simulink model "Model_10_1"  (R2021a)
settings: Solver=VariableStepAuto  StartTime=0.0  StopTime=10  RelTol=1e-3
InitFcn:
  | bx=25; %25
  | bl=50; %50
  | bc=0.1; %0.08
  | 
  | ml=2; %2
  | 
  | mc=0.5;
  | M2=0.5;
  | 
  | mt=5;
  | g=9.81;
  | l_ref=0.3; %0.3
  | l_ini=1;   %1
  | l=l_ini;
  | x_ref=1; %3
  | n1=1; %5
  | n2=1;
  | 
  | L_2=0;  %chieu dai day nang ha
  | 
  | theta1_ini=0*pi/180;
  | theta2_ini=0*pi/180;  %2*pi/180
  | 
  | L_tai=0.1;
  | %ADRC' s parameter caculation
  | %b0 = (1)/(mc+mt+ml);
  | b0=(ml+mc)/(mt*mc+2*ml*mc+mt*ml+ml^2+mc^2); %Enhanced-coupling
  | %k_ESO = 100;
  | k_ESO = 100;
  | T_set  = 3; %5;
  | 
  | s_cl = -5.85/T_set;
  | Kp   = s_cl^2;
  | Kd   = -2*s_cl;
  | 
  | s_ESO = k_ESO*s_cl;
  | l1        = -3*s_ESO;
  | l2        = 3*( s_ESO)^2;
  | l3        = -(s_ESO)^3;
  | 
  | %b1 = (mt+mc)/(mc*ml +mc*mt+ml*mt);
  | b1=1/(ml+mc);
  | k_ESO1 =100; %100
  | T_set1  = 3;   %3
  | s_cl1 = -5.85/T_set1;
  | Kp1   = s_cl1^2;
  | Kd1   = -2*s_cl1;
  | 
  | s_ESO1 = k_ESO1*s_cl1;
  | l11        = -3*s_ESO1;
  | l21        = 3*( s_ESO1)^2;
  | l31        = -(s_ESO1)^3;
  | 
  | 
  | %L1=l_ini;
  | L11=0.65;
  | L2=L_tai;
  | m1=2;
  | %m2=M2;
  | m=5;
  | ... (+35 lines)
libraries: neural x1372, simulink x44, simulink_extras x6
(part 2 of 58)

== system Model_10_1/26_12_theta1 bang 0 n1=5; n2=1 / ban đầu theta1=10pi//180, theta2=0_1 ==
  Fx : Inport
  Fl : Inport  Port=2
  Add : Sum
  Constant : Constant  Value=-(m1+mc)*g
  Constant1 : Constant  Value=mc
  Constant2 : Constant  Value=L_tai
  Crane : MATLAB Function  TreatAsAtomicUnit=on
  Integrator{,1,3,5..7} (6 alike) : Integrator
  Integrator2 : Integrator  InitialCondition=l
  Integrator4 : Integrator  InitialCondition=10*pi/180
  Scope{1..5} (5 alike) : Scope
  x : Outport
  l : Outport  Port=2
  the1 : Outport  Port=3
  the2 : Outport  Port=4
  wires:
  Integrator5/1 -> [x6]
  Integrator2/1 -> Scope4/1, l/1, [x3]
  Integrator1/1 -> [x2]
  Integrator/1 -> x/1, [x1]
  Integrator3/1 -> [x4]
  Add/1 -> Crane/9(Fl), Scope1/1
  Integrator6/1 -> Scope2/1, the2/1, [x7]
  Integrator7/1 -> [x8]
  Crane/1(dx1) -> Integrator/1
  Crane/2(dx2) -> Integrator1/1
  Crane/3(dx3) -> Integrator2/1
  Crane/4(dx4) -> Integrator3/1
  Crane/5(dx5) -> Integrator4/1
  Crane/6(dx6) -> Integrator5/1
  Crane/7(dx7) -> Integrator6/1
  Crane/8(dx8) -> Integrator7/1
  Fx/1 -> Crane/8(Fx)
  Constant1/1 -> Crane/10(m2)
  [x2] -> Crane/1(d1x)
  [x3] -> Crane/2(l1)
  [x4] -> Crane/3(d1l1)
  [x5] -> Crane/4(the1)
  [x6] -> Crane/5(d1the1)
  [x7] -> Crane/6(the2)
  [x8] -> Crane/7(d1the2)
  Integrator4/1 -> Scope3/1, the1/1, [x5]
  Fl/1 -> Add/2
  [x1] -> Scope5/1
  Constant/1 -> Add/1
  Constant2/1 -> Crane/11(l2)

== system Model_10_1/26_12_theta1 bang 0 n1=5; n2=1 /ADRC 1 ==
  ref : Inport
  x : Inport  Port=2
  Gain : Gain  Gain=Kp
  Gain1 : Gain  Gain=Kd
  Gain2 : Gain  Gain=1/b0
  Observer : Subsystem
  Sum : Sum  Inputs=|+-
  Sum3 : Sum  Inputs=|+-
  Sum4 : Sum  Inputs=|+-
  u : Outport
  wires:
  Sum4/1 -> Gain2/1
  Sum/1 -> Gain/1
  Gain2/1 -> u/1, Observer/1(u)
  x/1 -> Observer/2(x)
  Sum3/1 -> Sum4/1
  Observer/2(x2) -> Gain1/1
  Gain1/1 -> Sum3/2
  Gain/1 -> Sum3/1
  ref/1 -> Sum/1
  Observer/1(x3) -> Sum4/2
  Observer/3(x1) -> Sum/2

== system Model_10_1/26_12_theta1 bang 0 n1=5; n2=1 /ADRC 10 ==
  ref : Inport
  x : Inport  Port=2
  Gain : Gain  Gain=Kp
  Gain1 : Gain  Gain=Kd
  Gain2 : Gain  Gain=1/b0
  Observer : Subsystem
  Sum : Sum  Inputs=|+-
  Sum3 : Sum  Inputs=|+-
  Sum4 : Sum  Inputs=|+-
  u : Outport
  wires:
  Sum4/1 -> Gain2/1
  Sum/1 -> Gain/1
  Gain2/1 -> u/1, Observer/1(u)
  x/1 -> Observer/2(x)
  Sum3/1 -> Sum4/1
  Observer/2(x2) -> Gain1/1
  Gain1/1 -> Sum3/2
  Gain/1 -> Sum3/1
  ref/1 -> Sum/1
  Observer/1(x3) -> Sum4/2
  Observer/3(x1) -> Sum/2

== system Model_10_1/26_12_theta1 bang 0 n1=5; n2=1 /ADRC 11 ==
  ref : Inport
  x : Inport  Port=2
  Gain : Gain  Gain=Kp1
  Gain1 : Gain  Gain=Kd1
  Gain2 : Gain  Gain=1/b1
  Observer : Subsystem
  Sum : Sum  Inputs=|+-
  Sum3 : Sum  Inputs=|+-
  Sum4 : Sum  Inputs=|+-
  u : Outport
  wires:
  Sum4/1 -> Gain2/1
  Sum/1 -> Gain/1
  Gain2/1 -> u/1, Observer/1(u)
  x/1 -> Observer/2(x)
  Sum3/1 -> Sum4/1
  Observer/2(x2) -> Gain1/1
  Gain1/1 -> Sum3/2
  Gain/1 -> Sum3/1
  ref/1 -> Sum/1
  Observer/1(x3) -> Sum4/2
  Observer/3(x1) -> Sum/2

== system Model_10_1/26_12_theta1 bang 0 n1=5; n2=1 /ADRC 12 ==
  ref : Inport
  x : Inport  Port=2
  Gain : Gain  Gain=Kp1
  Gain1 : Gain  Gain=Kd1
  Gain2 : Gain  Gain=1/b1
  Observer : Subsystem
  Sum : Sum  Inputs=|+-
  Sum3 : Sum  Inputs=|+-
  Sum4 : Sum  Inputs=|+-
  u : Outport
  wires:
  Sum4/1 -> Gain2/1
  Sum/1 -> Gain/1
  Gain2/1 -> u/1, Observer/1(u)
  x/1 -> Observer/2(x)
  Sum3/1 -> Sum4/1
  Observer/2(x2) -> Gain1/1
  Gain1/1 -> Sum3/2
  Gain/1 -> Sum3/1
  ref/1 -> Sum/1
  Observer/1(x3) -> Sum4/2
  Observer/3(x1) -> Sum/2

== system Model_10_1/26_12_theta1 bang 0 n1=5; n2=1 /ADRC 13 ==
  ref : Inport
  x : Inport  Port=2
  Gain : Gain  Gain=Kp1
  Gain1 : Gain  Gain=Kd1
  Gain2 : Gain  Gain=1/b1
  Observer : Subsystem
  Sum : Sum  Inputs=|+-
  Sum3 : Sum  Inputs=|+-
  Sum4 : Sum  Inputs=|+-
  u : Outport
  wires:
  Sum4/1 -> Gain2/1
  Sum/1 -> Gain/1
  Gain2/1 -> u/1, Observer/1(u)
  x/1 -> Observer/2(x)
  Sum3/1 -> Sum4/1
  Observer/2(x2) -> Gain1/1
  Gain1/1 -> Sum3/2
  Gain/1 -> Sum3/1
  ref/1 -> Sum/1
  Observer/1(x3) -> Sum4/2
  Observer/3(x1) -> Sum/2

== system Model_10_1/26_12_theta1 bang 0 n1=5; n2=1 /ADRC 14 ==
  ref : Inport
  x : Inport  Port=2
  Gain : Gain  Gain=Kp
  Gain1 : Gain  Gain=Kd
  Gain2 : Gain  Gain=1/b0
  Observer : Subsystem
  Sum : Sum  Inputs=|+-
  Sum3 : Sum  Inputs=|+-
  Sum4 : Sum  Inputs=|+-
  u : Outport
  wires:
  Sum4/1 -> Gain2/1
  Sum/1 -> Gain/1
  Gain2/1 -> u/1, Observer/1(u)
  x/1 -> Observer/2(x)
  Sum3/1 -> Sum4/1
  Observer/2(x2) -> Gain1/1
  Gain1/1 -> Sum3/2
  Gain/1 -> Sum3/1
  ref/1 -> Sum/1
  Observer/1(x3) -> Sum4/2
  Observer/3(x1) -> Sum/2

== system Model_10_1/26_12_theta1 bang 0 n1=5; n2=1 /ADRC 17 ==
  ref : Inport
  x : Inport  Port=2
  Gain : Gain  Gain=Kp
  Gain1 : Gain  Gain=Kd
  Gain2 : Gain  Gain=1/b0
  Observer : Subsystem
  Sum : Sum  Inputs=|+-
  Sum3 : Sum  Inputs=|+-
  Sum4 : Sum  Inputs=|+-
  u : Outport
  wires:
  Sum4/1 -> Gain2/1
  Sum/1 -> Gain/1
  Gain2/1 -> u/1, Observer/1(u)
  x/1 -> Observer/2(x)
  Sum3/1 -> Sum4/1
  Observer/2(x2) -> Gain1/1
  Gain1/1 -> Sum3/2
  Gain/1 -> Sum3/1
  ref/1 -> Sum/1
  Observer/1(x3) -> Sum4/2
  Observer/3(x1) -> Sum/2

== system Model_10_1/26_12_theta1 bang 0 n1=5; n2=1 /ADRC 18 ==
  ref : Inport
  x : Inport  Port=2
  Gain : Gain  Gain=Kp1
  Gain1 : Gain  Gain=Kd1
  Gain2 : Gain  Gain=1/b1
  Observer : Subsystem
  Sum : Sum  Inputs=|+-
  Sum3 : Sum  Inputs=|+-
  Sum4 : Sum  Inputs=|+-
  u : Outport
  wires:
  Sum4/1 -> Gain2/1
  Sum/1 -> Gain/1
  Gain2/1 -> u/1, Observer/1(u)
  x/1 -> Observer/2(x)
  Sum3/1 -> Sum4/1
  Observer/2(x2) -> Gain1/1
  Gain1/1 -> Sum3/2
  Gain/1 -> Sum3/1
  ref/1 -> Sum/1
  Observer/1(x3) -> Sum4/2
  Observer/3(x1) -> Sum/2

== system Model_10_1/26_12_theta1 bang 0 n1=5; n2=1 /ADRC 19 ==
  ref : Inport
  x : Inport  Port=2
  Gain : Gain  Gain=Kp
  Gain1 : Gain  Gain=Kd
  Gain2 : Gain  Gain=1/b0
  Observer : Subsystem
  Sum : Sum  Inputs=|+-
  Sum3 : Sum  Inputs=|+-
  Sum4 : Sum  Inputs=|+-
  u : Outport
  wires:
  Sum4/1 -> Gain2/1
  Sum/1 -> Gain/1
  Gain2/1 -> u/1, Observer/1(u)
  x/1 -> Observer/2(x)
  Sum3/1 -> Sum4/1
  Observer/2(x2) -> Gain1/1
  Gain1/1 -> Sum3/2
  Gain/1 -> Sum3/1
  ref/1 -> Sum/1
  Observer/1(x3) -> Sum4/2
  Observer/3(x1) -> Sum/2

== system Model_10_1/26_12_theta1 bang 0 n1=5; n2=1 /ADRC 2 ==
  ref : Inport
  x : Inport  Port=2
  Gain : Gain  Gain=Kp1
  Gain1 : Gain  Gain=Kd1
  Gain2 : Gain  Gain=1/b1
  Observer : Subsystem
  Sum : Sum  Inputs=|+-
  Sum3 : Sum  Inputs=|+-
  Sum4 : Sum  Inputs=|+-
  u : Outport
  wires:
  Sum4/1 -> Gain2/1
  Sum/1 -> Gain/1
  Gain2/1 -> u/1, Observer/1(u)
  x/1 -> Observer/2(x)
  Sum3/1 -> Sum4/1
  Observer/2(x2) -> Gain1/1
  Gain1/1 -> Sum3/2
  Gain/1 -> Sum3/1
  ref/1 -> Sum/1
  Observer/1(x3) -> Sum4/2
  Observer/3(x1) -> Sum/2

== system Model_10_1/26_12_theta1 bang 0 n1=5; n2=1 /ADRC 20 ==
  ref : Inport
  x : Inport  Port=2
  Gain : Gain  Gain=Kp1
  Gain1 : Gain  Gain=Kd1
  Gain2 : Gain  Gain=1/b1
  Observer : Subsystem
  Sum : Sum  Inputs=|+-
  Sum3 : Sum  Inputs=|+-
  Sum4 : Sum  Inputs=|+-
  u : Outport
  wires:
  Sum4/1 -> Gain2/1
  Sum/1 -> Gain/1
  Gain2/1 -> u/1, Observer/1(u)
  x/1 -> Observer/2(x)
  Sum3/1 -> Sum4/1
  Observer/2(x2) -> Gain1/1
  Gain1/1 -> Sum3/2
  Gain/1 -> Sum3/1
  ref/1 -> Sum/1
  Observer/1(x3) -> Sum4/2
  Observer/3(x1) -> Sum/2

== system Model_10_1/26_12_theta1 bang 0 n1=5; n2=1 /ADRC 3 ==
  ref : Inport
  x : Inport  Port=2
  Gain : Gain  Gain=Kp
  Gain1 : Gain  Gain=Kd
  Gain2 : Gain  Gain=1/b0
  Observer : Subsystem
  Sum : Sum  Inputs=|+-
  Sum3 : Sum  Inputs=|+-
  Sum4 : Sum  Inputs=|+-
  u : Outport
  wires:
  Sum4/1 -> Gain2/1
  Sum/1 -> Gain/1
  Gain2/1 -> u/1, Observer/1(u)
  x/1 -> Observer/2(x)
  Sum3/1 -> Sum4/1
  Observer/2(x2) -> Gain1/1
  Gain1/1 -> Sum3/2
  Gain/1 -> Sum3/1
  ref/1 -> Sum/1
  Observer/1(x3) -> Sum4/2
  Observer/3(x1) -> Sum/2

== system Model_10_1/26_12_theta1 bang 0 n1=5; n2=1 /ADRC 4 ==
  ref : Inport
  x : Inport  Port=2
  Gain : Gain  Gain=Kp1
  Gain1 : Gain  Gain=Kd1
  Gain2 : Gain  Gain=1/b1
  Observer : Subsystem
  Sum : Sum  Inputs=|+-
  Sum3 : Sum  Inputs=|+-
  Sum4 : Sum  Inputs=|+-
  u : Outport
  wires:
  Sum4/1 -> Gain2/1
  Sum/1 -> Gain/1
  Gain2/1 -> u/1, Observer/1(u)
  x/1 -> Observer/2(x)
  Sum3/1 -> Sum4/1
  Observer/2(x2) -> Gain1/1
  Gain1/1 -> Sum3/2
  Gain/1 -> Sum3/1
  ref/1 -> Sum/1
  Observer/1(x3) -> Sum4/2
  Observer/3(x1) -> Sum/2

== system Model_10_1/26_12_theta1 bang 0 n1=5; n2=1 /ADRC 9 ==
  ref : Inport
  x : Inport  Port=2
  Gain : Gain  Gain=Kp
  Gain1 : Gain  Gain=Kd
  Gain2 : Gain  Gain=1/b0
  Observer : Subsystem
  Sum : Sum  Inputs=|+-
  Sum3 : Sum  Inputs=|+-
  Sum4 : Sum  Inputs=|+-
  u : Outport
  wires:
  Sum4/1 -> Gain2/1
  Sum/1 -> Gain/1
  Gain2/1 -> u/1, Observer/1(u)
  x/1 -> Observer/2(x)
  Sum3/1 -> Sum4/1
  Observer/2(x2) -> Gain1/1
  Gain1/1 -> Sum3/2
  Gain/1 -> Sum3/1
  ref/1 -> Sum/1
  Observer/1(x3) -> Sum4/2
  Observer/3(x1) -> Sum/2

== system Model_10_1/26_12_theta1 bang 0 n1=5; n2=1 /Bo1_LT_L2=0.1_2 ==
  Input : Inport  PortDimensions=2
      mask Display: e = 0.06;c1 = [120 230 180]/255;c2 = ([120 230 180]+0)/(256+128);c3 = ([120 230 180]+128)/(256+128);patch([0 1 1 0],[0 0 1 1],c1);patch([0 1 1 1-e 1-e 0+e],[0 0 1 1-e 0+e 0+e],c2);patch([0 0 1 1-e 0+e 0+e],[0 1 1 1-e 1-e 0+e],c3);plot([0 1 1 0 0],[0 0 1 1 0]);
  Layer 1 : Subsystem
      mask Display: e = 0.06;c1 = [120 150 230]/255;c2 = ([120 150 230]+0)/383;c3 = ([120 150 230]+128)/383;patch([0 1 1 0],[0 0 1 1],c1);patch([0 1 1 1-e 1-e 0+e],[0 0 1 1-e 0+e 0+e],c2);patch([0 0 1 1-e 0+e 0+e],[0 1 1 1-e 1-e 0+e],c3);plot([0 1 1 0 0],[0 0 1 1 0]);
  Layer 2 : Subsystem
      mask Display: e = 0.06;c1 = [120 150 230]/255;c2 = ([120 150 230]+0)/383;c3 = ([120 150 230]+128)/383;patch([0 1 1 0],[0 0 1 1],c1);patch([0 1 1 1-e 1-e 0+e],[0 0 1 1-e 0+e 0+e],c2);patch([0 0 1 1-e 0+e 0+e],[0 1 1 1-e 1-e 0+e],c3);plot([0 1 1 0 0],[0 0 1 1 0]);
  Process Input 1 : Subsystem
      mask Display: e = 0.06;c1 = [120 150 230]/255;c2 = ([120 150 230]+0)/383;c3 = ([120 150 230]+128)/383;patch([0 1 1 0],[0 0 1 1],c1);patch([0 1 1 1-e 1-e 0+e],[0 0 1 1-e 0+e 0+e],c2);patch([0 0 1 1-e 0+e 0+e],[0 1 1 1-e 1-e 0+e],c3);plot([0 1 1 0 0],[0 0 1 1 0]);
  Process Output 1 : Subsystem
      mask Display: e = 0.06;c1 = [120 150 230]/255;c2 = ([120 150 230]+0)/383;c3 = ([120 150 230]+128)/383;patch([0 1 1 0],[0 0 1 1],c1);patch([0 1 1 1-e 1-e 0+e],[0 0 1 1-e 0+e 0+e],c2);patch([0 0 1 1-e 0+e 0+e],[0 1 1 1-e 1-e 0+e],c3);plot([0 1 1 0 0],[0 0 1 1 0]);
  Output : Outport  InitialOutput=[0;0;0]
      mask Display: e = 0.06;c1 = [120 230 180]/255;c2 = ([120 230 180]+0)/(256+128);c3 = ([120 230 180]+128)/(256+128);patch([0 1 1 0],[0 0 1 1],c1);patch([0 1 1 1-e 1-e 0+e],[0 0 1 1-e 0+e 0+e],c2);patch([0 0 1 1-e 0+e 0+e],[0 1 1 1-e 1-e 0+e],c3);plot([0 1 1 0 0],[0 0 1 1 0]);
  wires:
  Input/1 -> Process Input 1/1(x)
  Process Output 1/1(y) -> Output/1
  Process Input 1/1(p) -> Layer 1/1("p{1}")
  Layer 1/1("a{1}") -> [feedback1]
  [feedback1] -> Layer 2/1("a{1} ")
  Layer 2/1("a{2}") -> Process Output 1/1(a)

== system Model_10_1/26_12_theta1 bang 0 n1=5; n2=1 /Bo1_LT_L2=0.1_3 ==
  Input : Inport  PortDimensions=2
      mask Display: e = 0.06;c1 = [120 230 180]/255;c2 = ([120 230 180]+0)/(256+128);c3 = ([120 230 180]+128)/(256+128);patch([0 1 1 0],[0 0 1 1],c1);patch([0 1 1 1-e 1-e 0+e],[0 0 1 1-e 0+e 0+e],c2);patch([0 0 1 1-e 0+e 0+e],[0 1 1 1-e 1-e 0+e],c3);plot([0 1 1 0 0],[0 0 1 1 0]);
  Layer 1 : Subsystem
      mask Display: e = 0.06;c1 = [120 150 230]/255;c2 = ([120 150 230]+0)/383;c3 = ([120 150 230]+128)/383;patch([0 1 1 0],[0 0 1 1],c1);patch([0 1 1 1-e 1-e 0+e],[0 0 1 1-e 0+e 0+e],c2);patch([0 0 1 1-e 0+e 0+e],[0 1 1 1-e 1-e 0+e],c3);plot([0 1 1 0 0],[0 0 1 1 0]);
  Layer 2 : Subsystem
      mask Display: e = 0.06;c1 = [120 150 230]/255;c2 = ([120 150 230]+0)/383;c3 = ([120 150 230]+128)/383;patch([0 1 1 0],[0 0 1 1],c1);patch([0 1 1 1-e 1-e 0+e],[0 0 1 1-e 0+e 0+e],c2);patch([0 0 1 1-e 0+e 0+e],[0 1 1 1-e 1-e 0+e],c3);plot([0 1 1 0 0],[0 0 1 1 0]);
  Process Input 1 : Subsystem
      mask Display: e = 0.06;c1 = [120 150 230]/255;c2 = ([120 150 230]+0)/383;c3 = ([120 150 230]+128)/383;patch([0 1 1 0],[0 0 1 1],c1);patch([0 1 1 1-e 1-e 0+e],[0 0 1 1-e 0+e 0+e],c2);patch([0 0 1 1-e 0+e 0+e],[0 1 1 1-e 1-e 0+e],c3);plot([0 1 1 0 0],[0 0 1 1 0]);
  Process Output 1 : Subsystem
      mask Display: e = 0.06;c1 = [120 150 230]/255;c2 = ([120 150 230]+0)/383;c3 = ([120 150 230]+128)/383;patch([0 1 1 0],[0 0 1 1],c1);patch([0 1 1 1-e 1-e 0+e],[0 0 1 1-e 0+e 0+e],c2);patch([0 0 1 1-e 0+e 0+e],[0 1 1 1-e 1-e 0+e],c3);plot([0 1 1 0 0],[0 0 1 1 0]);
  Output : Outport  InitialOutput=[0;0;0]
      mask Display: e = 0.06;c1 = [120 230 180]/255;c2 = ([120 230 180]+0)/(256+128);c3 = ([120 230 180]+128)/(256+128);patch([0 1 1 0],[0 0 1 1],c1);patch([0 1 1 1-e 1-e 0+e],[0 0 1 1-e 0+e 0+e],c2);patch([0 0 1 1-e 0+e 0+e],[0 1 1 1-e 1-e 0+e],c3);plot([0 1 1 0 0],[0 0 1 1 0]);
  wires:
  Input/1 -> Process Input 1/1(x)
  Process Output 1/1(y) -> Output/1
  Process Input 1/1(p) -> Layer 1/1("p{1}")
  Layer 1/1("a{1}") -> [feedback1]
  [feedback1] -> Layer 2/1("a{1} ")
  Layer 2/1("a{2}") -> Process Output 1/1(a)

== system Model_10_1/26_12_theta1 bang 0 n1=5; n2=1 /Bo2_LT_L2=0.1 ==
  Input : Inport  PortDimensions=2
      mask Display: e = 0.06;c1 = [120 230 180]/255;c2 = ([120 230 180]+0)/(256+128);c3 = ([120 230 180]+128)/(256+128);patch([0 1 1 0],[0 0 1 1],c1);patch([0 1 1 1-e 1-e 0+e],[0 0 1 1-e 0+e 0+e],c2);patch([0 0 1 1-e 0+e 0+e],[0 1 1 1-e 1-e 0+e],c3);plot([0 1 1 0 0],[0 0 1 1 0]);
  Layer 1 : Subsystem
      mask Display: e = 0.06;c1 = [120 150 230]/255;c2 = ([120 150 230]+0)/383;c3 = ([120 150 230]+128)/383;patch([0 1 1 0],[0 0 1 1],c1);patch([0 1 1 1-e 1-e 0+e],[0 0 1 1-e 0+e 0+e],c2);patch([0 0 1 1-e 0+e 0+e],[0 1 1 1-e 1-e 0+e],c3);plot([0 1 1 0 0],[0 0 1 1 0]);
  Layer 2 : Subsystem
      mask Display: e = 0.06;c1 = [120 150 230]/255;c2 = ([120 150 230]+0)/383;c3 = ([120 150 230]+128)/383;patch([0 1 1 0],[0 0 1 1],c1);patch([0 1 1 1-e 1-e 0+e],[0 0 1 1-e 0+e 0+e],c2);patch([0 0 1 1-e 0+e 0+e],[0 1 1 1-e 1-e 0+e],c3);plot([0 1 1 0 0],[0 0 1 1 0]);
  Process Input 1 : Subsystem
      mask Display: e = 0.06;c1 = [120 150 230]/255;c2 = ([120 150 230]+0)/383;c3 = ([120 150 230]+128)/383;patch([0 1 1 0],[0 0 1 1],c1);patch([0 1 1 1-e 1-e 0+e],[0 0 1 1-e 0+e 0+e],c2);patch([0 0 1 1-e 0+e 0+e],[0 1 1 1-e 1-e 0+e],c3);plot([0 1 1 0 0],[0 0 1 1 0]);
  Process Output 1 : Subsystem
      mask Display: e = 0.06;c1 = [120 150 230]/255;c2 = ([120 150 230]+0)/383;c3 = ([120 150 230]+128)/383;patch([0 1 1 0],[0 0 1 1],c1);patch([0 1 1 1-e 1-e 0+e],[0 0 1 1-e 0+e 0+e],c2);patch([0 0 1 1-e 0+e 0+e],[0 1 1 1-e 1-e 0+e],c3);plot([0 1 1 0 0],[0 0 1 1 0]);
  Output : Outport  InitialOutput=[0;0;0]
      mask Display: e = 0.06;c1 = [120 230 180]/255;c2 = ([120 230 180]+0)/(256+128);c3 = ([120 230 180]+128)/(256+128);patch([0 1 1 0],[0 0 1 1],c1);patch([0 1 1 1-e 1-e 0+e],[0 0 1 1-e 0+e 0+e],c2);patch([0 0 1 1-e 0+e 0+e],[0 1 1 1-e 1-e 0+e],c3);plot([0 1 1 0 0],[0 0 1 1 0]);
  wires:
  Input/1 -> Process Input 1/1(x)
  Process Output 1/1(y) -> Output/1
  Process Input 1/1(p) -> Layer 1/1("p{1}")
  Layer 1/1("a{1}") -> [feedback1]
  [feedback1] -> Layer 2/1("a{1} ")
  Layer 2/1("a{2}") -> Process Output 1/1(a)

== system Model_10_1/26_12_theta1 bang 0 n1=5; n2=1 /Bo2_LT_L2=0.1_2 ==
  Input : Inport  PortDimensions=2
      mask Display: e = 0.06;c1 = [120 230 180]/255;c2 = ([120 230 180]+0)/(256+128);c3 = ([120 230 180]+128)/(256+128);patch([0 1 1 0],[0 0 1 1],c1);patch([0 1 1 1-e 1-e 0+e],[0 0 1 1-e 0+e 0+e],c2);patch([0 0 1 1-e 0+e 0+e],[0 1 1 1-e 1-e 0+e],c3);plot([0 1 1 0 0],[0 0 1 1 0]);
  Layer 1 : Subsystem
      mask Display: e = 0.06;c1 = [120 150 230]/255;c2 = ([120 150 230]+0)/383;c3 = ([120 150 230]+128)/383;patch([0 1 1 0],[0 0 1 1],c1);patch([0 1 1 1-e 1-e 0+e],[0 0 1 1-e 0+e 0+e],c2);patch([0 0 1 1-e 0+e 0+e],[0 1 1 1-e 1-e 0+e],c3);plot([0 1 1 0 0],[0 0 1 1 0]);
  Layer 2 : Subsystem
      mask Display: e = 0.06;c1 = [120 150 230]/255;c2 = ([120 150 230]+0)/383;c3 = ([120 150 230]+128)/383;patch([0 1 1 0],[0 0 1 1],c1);patch([0 1 1 1-e 1-e 0+e],[0 0 1 1-e 0+e 0+e],c2);patch([0 0 1 1-e 0+e 0+e],[0 1 1 1-e 1-e 0+e],c3);plot([0 1 1 0 0],[0 0 1 1 0]);
  Process Input 1 : Subsystem
      mask Display: e = 0.06;c1 = [120 150 230]/255;c2 = ([120 150 230]+0)/383;c3 = ([120 150 230]+128)/383;patch([0 1 1 0],[0 0 1 1],c1);patch([0 1 1 1-e 1-e 0+e],[0 0 1 1-e 0+e 0+e],c2);patch([0 0 1 1-e 0+e 0+e],[0 1 1 1-e 1-e 0+e],c3);plot([0 1 1 0 0],[0 0 1 1 0]);
  Process Output 1 : Subsystem
      mask Display: e = 0.06;c1 = [120 150 230]/255;c2 = ([120 150 230]+0)/383;c3 = ([120 150 230]+128)/383;patch([0 1 1 0],[0 0 1 1],c1);patch([0 1 1 1-e 1-e 0+e],[0 0 1 1-e 0+e 0+e],c2);patch([0 0 1 1-e 0+e 0+e],[0 1 1 1-e 1-e 0+e],c3);plot([0 1 1 0 0],[0 0 1 1 0]);
  Output : Outport  InitialOutput=[0;0;0]
      mask Display: e = 0.06;c1 = [120 230 180]/255;c2 = ([120 230 180]+0)/(256+128);c3 = ([120 230 180]+128)/(256+128);patch([0 1 1 0],[0 0 1 1],c1);patch([0 1 1 1-e 1-e 0+e],[0 0 1 1-e 0+e 0+e],c2);patch([0 0 1 1-e 0+e 0+e],[0 1 1 1-e 1-e 0+e],c3);plot([0 1 1 0 0],[0 0 1 1 0]);
  wires:
  Input/1 -> Process Input 1/1(x)
  Process Output 1/1(y) -> Output/1
  Process Input 1/1(p) -> Layer 1/1("p{1}")
  Layer 1/1("a{1}") -> [feedback1]
  [feedback1] -> Layer 2/1("a{1} ")
  Layer 2/1("a{2}") -> Process Output 1/1(a)

== system Model_10_1/26_12_theta1 bang 0 n1=5; n2=1 /Bo2_LT_L2=0.3 ==
  Input : Inport  PortDimensions=2
      mask Display: e = 0.06;c1 = [120 230 180]/255;c2 = ([120 230 180]+0)/(256+128);c3 = ([120 230 180]+128)/(256+128);patch([0 1 1 0],[0 0 1 1],c1);patch([0 1 1 1-e 1-e 0+e],[0 0 1 1-e 0+e 0+e],c2);patch([0 0 1 1-e 0+e 0+e],[0 1 1 1-e 1-e 0+e],c3);plot([0 1 1 0 0],[0 0 1 1 0]);
  Layer 1 : Subsystem
      mask Display: e = 0.06;c1 = [120 150 230]/255;c2 = ([120 150 230]+0)/383;c3 = ([120 150 230]+128)/383;patch([0 1 1 0],[0 0 1 1],c1);patch([0 1 1 1-e 1-e 0+e],[0 0 1 1-e 0+e 0+e],c2);patch([0 0 1 1-e 0+e 0+e],[0 1 1 1-e 1-e 0+e],c3);plot([0 1 1 0 0],[0 0 1 1 0]);
  Layer 2 : Subsystem
      mask Display: e = 0.06;c1 = [120 150 230]/255;c2 = ([120 150 230]+0)/383;c3 = ([120 150 230]+128)/383;patch([0 1 1 0],[0 0 1 1],c1);patch([0 1 1 1-e 1-e 0+e],[0 0 1 1-e 0+e 0+e],c2);patch([0 0 1 1-e 0+e 0+e],[0 1 1 1-e 1-e 0+e],c3);plot([0 1 1 0 0],[0 0 1 1 0]);
  Process Input 1 : Subsystem
      mask Display: e = 0.06;c1 = [120 150 230]/255;c2 = ([120 150 230]+0)/383;c3 = ([120 150 230]+128)/383;patch([0 1 1 0],[0 0 1 1],c1);patch([0 1 1 1-e 1-e 0+e],[0 0 1 1-e 0+e 0+e],c2);patch([0 0 1 1-e 0+e 0+e],[0 1 1 1-e 1-e 0+e],c3);plot([0 1 1 0 0],[0 0 1 1 0]);
  Process Output 1 : Subsystem
      mask Display: e = 0.06;c1 = [120 150 230]/255;c2 = ([120 150 230]+0)/383;c3 = ([120 150 230]+128)/383;patch([0 1 1 0],[0 0 1 1],c1);patch([0 1 1 1-e 1-e 0+e],[0 0 1 1-e 0+e 0+e],c2);patch([0 0 1 1-e 0+e 0+e],[0 1 1 1-e 1-e 0+e],c3);plot([0 1 1 0 0],[0 0 1 1 0]);
  Output : Outport  InitialOutput=[0;0;0]
      mask Display: e = 0.06;c1 = [120 230 180]/255;c2 = ([120 230 180]+0)/(256+128);c3 = ([120 230 180]+128)/(256+128);patch([0 1 1 0],[0 0 1 1],c1);patch([0 1 1 1-e 1-e 0+e],[0 0 1 1-e 0+e 0+e],c2);patch([0 0 1 1-e 0+e 0+e],[0 1 1 1-e 1-e 0+e],c3);plot([0 1 1 0 0],[0 0 1 1 0]);
  wires:
  Input/1 -> Process Input 1/1(x)
  Process Output 1/1(y) -> Output/1
  Process Input 1/1(p) -> Layer 1/1("p{1}")
  Layer 1/1("a{1}") -> [feedback1]
  [feedback1] -> Layer 2/1("a{1} ")
  Layer 2/1("a{2}") -> Process Output 1/1(a)

== system Model_10_1/26_12_theta1 bang 0 n1=5; n2=1 /Co FL_25.12 ==
  Input : Inport  PortDimensions=2
      mask Display: e = 0.06;c1 = [120 230 180]/255;c2 = ([120 230 180]+0)/(256+128);c3 = ([120 230 180]+128)/(256+128);patch([0 1 1 0],[0 0 1 1],c1);patch([0 1 1 1-e 1-e 0+e],[0 0 1 1-e 0+e 0+e],c2);patch([0 0 1 1-e 0+e 0+e],[0 1 1 1-e 1-e 0+e],c3);plot([0 1 1 0 0],[0 0 1 1 0]);
  Layer 1 : Subsystem
      mask Display: e = 0.06;c1 = [120 150 230]/255;c2 = ([120 150 230]+0)/383;c3 = ([120 150 230]+128)/383;patch([0 1 1 0],[0 0 1 1],c1);patch([0 1 1 1-e 1-e 0+e],[0 0 1 1-e 0+e 0+e],c2);patch([0 0 1 1-e 0+e 0+e],[0 1 1 1-e 1-e 0+e],c3);plot([0 1 1 0 0],[0 0 1 1 0]);
  Layer 2 : Subsystem
      mask Display: e = 0.06;c1 = [120 150 230]/255;c2 = ([120 150 230]+0)/383;c3 = ([120 150 230]+128)/383;patch([0 1 1 0],[0 0 1 1],c1);patch([0 1 1 1-e 1-e 0+e],[0 0 1 1-e 0+e 0+e],c2);patch([0 0 1 1-e 0+e 0+e],[0 1 1 1-e 1-e 0+e],c3);plot([0 1 1 0 0],[0 0 1 1 0]);
  Process Input 1 : Subsystem
      mask Display: e = 0.06;c1 = [120 150 230]/255;c2 = ([120 150 230]+0)/383;c3 = ([120 150 230]+128)/383;patch([0 1 1 0],[0 0 1 1],c1);patch([0 1 1 1-e 1-e 0+e],[0 0 1 1-e 0+e 0+e],c2);patch([0 0 1 1-e 0+e 0+e],[0 1 1 1-e 1-e 0+e],c3);plot([0 1 1 0 0],[0 0 1 1 0]);
  Process Output 1 : Subsystem
      mask Display: e = 0.06;c1 = [120 150 230]/255;c2 = ([120 150 230]+0)/383;c3 = ([120 150 230]+128)/383;patch([0 1 1 0],[0 0 1 1],c1);patch([0 1 1 1-e 1-e 0+e],[0 0 1 1-e 0+e 0+e],c2);patch([0 0 1 1-e 0+e 0+e],[0 1 1 1-e 1-e 0+e],c3);plot([0 1 1 0 0],[0 0 1 1 0]);
  Output : Outport  InitialOutput=[0;0;0]
      mask Display: e = 0.06;c1 = [120 230 180]/255;c2 = ([120 230 180]+0)/(256+128);c3 = ([120 230 180]+128)/(256+128);patch([0 1 1 0],[0 0 1 1],c1);patch([0 1 1 1-e 1-e 0+e],[0 0 1 1-e 0+e 0+e],c2);patch([0 0 1 1-e 0+e 0+e],[0 1 1 1-e 1-e 0+e],c3);plot([0 1 1 0 0],[0 0 1 1 0]);
  wires:
  Input/1 -> Process Input 1/1(x)
  Process Output 1/1(y) -> Output/1
  Process Input 1/1(p) -> Layer 1/1("p{1}")
  Layer 1/1("a{1}") -> [feedback1]
  [feedback1] -> Layer 2/1("a{1} ")
  Layer 2/1("a{2}") -> Process Output 1/1(a)

== system Model_10_1/26_12_theta1 bang 0 n1=5; n2=1 /ETM2 ==
  ref_ETm4 : Inport
  ETM1 : Subsystem
  ETM4 : Subsystem
  ref1 : Scope
  ref2 : Scope
  ref3 : Scope
  ref_ETM4 : Outport
  wires:
  ETM1/1(Out1) -> ref2/1, ETM4/1(In1)  "ref_ZV"
  ETM4/1(Out1) -> ref3/1, ref_ETM4/1  "ref_ZV"
  ref_ETm4/1 -> ref1/1, ETM1/1(In1)

== system Model_10_1/26_12_theta1 bang 0 n1=5; n2=1 /Fl bo 1 (2 5 3) (2) ==
  Input : Inport  PortDimensions=2
      mask Display: e = 0.06;c1 = [120 230 180]/255;c2 = ([120 230 180]+0)/(256+128);c3 = ([120 230 180]+128)/(256+128);patch([0 1 1 0],[0 0 1 1],c1);patch([0 1 1 1-e 1-e 0+e],[0 0 1 1-e 0+e 0+e],c2);patch([0 0 1 1-e 0+e 0+e],[0 1 1 1-e 1-e 0+e],c3);plot([0 1 1 0 0],[0 0 1 1 0]);
  Layer 1 : Subsystem
      mask Display: e = 0.06;c1 = [120 150 230]/255;c2 = ([120 150 230]+0)/383;c3 = ([120 150 230]+128)/383;patch([0 1 1 0],[0 0 1 1],c1);patch([0 1 1 1-e 1-e 0+e],[0 0 1 1-e 0+e 0+e],c2);patch([0 0 1 1-e 0+e 0+e],[0 1 1 1-e 1-e 0+e],c3);plot([0 1 1 0 0],[0 0 1 1 0]);
  Layer 2 : Subsystem
      mask Display: e = 0.06;c1 = [120 150 230]/255;c2 = ([120 150 230]+0)/383;c3 = ([120 150 230]+128)/383;patch([0 1 1 0],[0 0 1 1],c1);patch([0 1 1 1-e 1-e 0+e],[0 0 1 1-e 0+e 0+e],c2);patch([0 0 1 1-e 0+e 0+e],[0 1 1 1-e 1-e 0+e],c3);plot([0 1 1 0 0],[0 0 1 1 0]);
  Process Input 1 : Subsystem
      mask Display: e = 0.06;c1 = [120 150 230]/255;c2 = ([120 150 230]+0)/383;c3 = ([120 150 230]+128)/383;patch([0 1 1 0],[0 0 1 1],c1);patch([0 1 1 1-e 1-e 0+e],[0 0 1 1-e 0+e 0+e],c2);patch([0 0 1 1-e 0+e 0+e],[0 1 1 1-e 1-e 0+e],c3);plot([0 1 1 0 0],[0 0 1 1 0]);
  Process Output 1 : Subsystem
      mask Display: e = 0.06;c1 = [120 150 230]/255;c2 = ([120 150 230]+0)/383;c3 = ([120 150 230]+128)/383;patch([0 1 1 0],[0 0 1 1],c1);patch([0 1 1 1-e 1-e 0+e],[0 0 1 1-e 0+e 0+e],c2);patch([0 0 1 1-e 0+e 0+e],[0 1 1 1-e 1-e 0+e],c3);plot([0 1 1 0 0],[0 0 1 1 0]);
  Output : Outport  InitialOutput=[0;0;0]
      mask Display: e = 0.06;c1 = [120 230 180]/255;c2 = ([120 230 180]+0)/(256+128);c3 = ([120 230 180]+128)/(256+128);patch([0 1 1 0],[0 0 1 1],c1);patch([0 1 1 1-e 1-e 0+e],[0 0 1 1-e 0+e 0+e],c2);patch([0 0 1 1-e 0+e 0+e],[0 1 1 1-e 1-e 0+e],c3);plot([0 1 1 0 0],[0 0 1 1 0]);
  wires:
  Input/1 -> Process Input 1/1(x)
  Process Output 1/1(y) -> Output/1
  Process Input 1/1(p) -> Layer 1/1("p{1}")
  Layer 1/1("a{1}") -> [feedback1]
  [feedback1] -> Layer 2/1("a{1} ")
  Layer 2/1("a{2}") -> Process Output 1/1(a)

== system Model_10_1/26_12_theta1 bang 0 n1=5; n2=1 /L_ref1 ==
  Add : Sum
  Step22 : Step  Time=0  Before=l_ini  After=l_ref  SampleTime=0
  Step23 : Step  Time=3  After=L_2  SampleTime=0
  out : Outport
  wires:
  Step23/1 -> Add/2  "ref_L"
  Add/1 -> out/1
  Step22/1 -> Add/1  "ref_L"

== system Model_10_1/26_12_theta1 bang 0 n1=5; n2=1 /L_ref2 ==
  Add : Sum
  Step22 : Step  Time=0  Before=l_ini  After=l_ref  SampleTime=0
  Step23 : Step  Time=3  After=L_2  SampleTime=0
  out : Outport
  wires:
  Step23/1 -> Add/2  "ref_L"
  Add/1 -> out/1
  Step22/1 -> Add/1  "ref_L"

== system Model_10_1/26_12_theta1 bang 0 n1=5; n2=1 /L_ref3 ==
  Add : Sum
  Step22 : Step  Time=0  Before=l_ini  After=l_ref  SampleTime=0
  Step23 : Step  Time=3  After=L_2  SampleTime=0
  out : Outport
  wires:
  Step23/1 -> Add/2  "ref_L"
  Add/1 -> out/1
  Step22/1 -> Add/1  "ref_L"

== system Model_10_1/26_12_theta1 bang 0 n1=5; n2=1 /L_ref4 ==
  Add : Sum
  Step22 : Step  Time=0  Before=l_ini  After=l_ref  SampleTime=0
  Step23 : Step  Time=3  After=L_2  SampleTime=0
  out : Outport
  wires:
  Step23/1 -> Add/2  "ref_L"
  Add/1 -> out/1
  Step22/1 -> Add/1  "ref_L"

== system Model_10_1/26_12_theta1 bang 0 n1=5; n2=1 /L_ref5 ==
  Add : Sum
  Step22 : Step  Time=0  Before=l_ini  After=l_ref  SampleTime=0
  Step23 : Step  Time=3  After=L_2  SampleTime=0
  out : Outport
  wires:
  Step23/1 -> Add/2  "ref_L"
  Add/1 -> out/1
  Step22/1 -> Add/1  "ref_L"

== system Model_10_1/26_12_theta1 bang 0 n1=5; n2=1 /L_ref6 ==
  Add : Sum
  Step22 : Step  Time=0  Before=l_ini  After=l_ref  SampleTime=0
  Step23 : Step  Time=3  After=L_2  SampleTime=0
  out : Outport
  wires:
  Step23/1 -> Add/2  "ref_L"
  Add/1 -> out/1
  Step22/1 -> Add/1  "ref_L"

== system Model_10_1/26_12_theta1 bang 0 n1=5; n2=1 /L_ref8 ==
  Add : Sum
  Step22 : Step  Time=0  Before=l_ini  After=l_ref  SampleTime=0
  Step23 : Step  Time=3  After=L_2  SampleTime=0
  out : Outport
  wires:
  Step23/1 -> Add/2  "ref_L"
  Add/1 -> out/1
  Step22/1 -> Add/1  "ref_L"

== system Model_10_1/26_12_theta1 bang 0 n1=5; n2=1 /PSO-ETM1 ==
  In1 : Inport
  Input : Inport  Port=2
  Input1 : Inport  Port=3
  Input2 : Inport  Port=4
  Gain : Gain  Gain=A1_etm4_2
  Gain1 : Gain  Gain=A2_etm4_2
  Gain2 : Gain  Gain=A3_etm4_2
  Gain3 : Gain  Gain=A4_etm4_2
  Sum : Sum  Inputs=++++
  Variable Transport Delay : VariableTransportDelay  VariableDelayType=Variable transport delay  MaximumDelay=10
  Variable Transport Delay1 : VariableTransportDelay  VariableDelayType=Variable transport delay  MaximumDelay=10
  Variable Transport Delay2 : VariableTransportDelay  VariableDelayType=Variable transport delay  MaximumDelay=10
  ref : Outport
  wires:
  In1/1 -> Gain1/1, Gain3/1, Gain2/1, Gain/1
  Gain1/1 -> Variable Transport Delay/1
  Variable Transport Delay/1 -> Sum/2
  Sum/1 -> ref/1
  Gain2/1 -> Variable Transport Delay1/1
  Gain/1 -> Sum/1
  Variable Transport Delay1/1 -> Sum/3
  Gain3/1 -> Variable Transport Delay2/1
  Variable Transport Delay2/1 -> Sum/4
  Input/1 -> Variable Transport Delay/2
  Input1/1 -> Variable Transport Delay1/2
  Input2/1 -> Variable Transport Delay2/2

== system Model_10_1/26_12_theta1 bang 0 n1=5; n2=1 /PSO-ETM2 ==
  In1 : Inport
  Input : Inport  Port=2
  Input1 : Inport  Port=3
  Input2 : Inport  Port=4
  Gain : Gain  Gain=0.1667
  Gain1 : Gain  Gain=0.3333
  Gain2 : Gain  Gain=0.3333
  Gain3 : Gain  Gain=0.1667
  Sum : Sum  Inputs=++++
  Variable Transport Delay : VariableTransportDelay  VariableDelayType=Variable transport delay  MaximumDelay=10
  Variable Transport Delay1 : VariableTransportDelay  VariableDelayType=Variable transport delay  MaximumDelay=10
  Variable Transport Delay2 : VariableTransportDelay  VariableDelayType=Variable transport delay  MaximumDelay=10
  ref : Outport
  wires:
  In1/1 -> Gain1/1, Gain3/1, Gain2/1, Gain/1
  Gain1/1 -> Variable Transport Delay/1
  Variable Transport Delay/1 -> Sum/2
  Sum/1 -> ref/1
  Gain2/1 -> Variable Transport Delay1/1
  Gain/1 -> Sum/1
  Variable Transport Delay1/1 -> Sum/3
  Gain3/1 -> Variable Transport Delay2/1
  Variable Transport Delay2/1 -> Sum/4
  Input/1 -> Variable Transport Delay/2
  Input1/1 -> Variable Transport Delay1/2
  Input2/1 -> Variable Transport Delay2/2

== system Model_10_1/26_12_theta1 bang 0 n1=5; n2=1 /PSO-ETM3 ==
  In1 : Inport
  Input : Inport  Port=2
  Input1 : Inport  Port=3
  Input2 : Inport  Port=4
  Gain : Gain  Gain=0.1667
  Gain1 : Gain  Gain=0.3333
  Gain2 : Gain  Gain=0.3333
  Gain3 : Gain  Gain=0.1667
  Sum : Sum  Inputs=++++
  Variable Transport Delay : VariableTransportDelay  VariableDelayType=Variable transport delay  MaximumDelay=10
  Variable Transport Delay1 : VariableTransportDelay  VariableDelayType=Variable transport delay  MaximumDelay=10
  Variable Transport Delay2 : VariableTransportDelay  VariableDelayType=Variable transport delay  MaximumDelay=10
  ref : Outport
  wires:
  In1/1 -> Gain1/1, Gain3/1, Gain2/1, Gain/1
  Gain1/1 -> Variable Transport Delay/1
  Variable Transport Delay/1 -> Sum/2
  Sum/1 -> ref/1
  Gain2/1 -> Variable Transport Delay1/1
  Gain/1 -> Sum/1
  Variable Transport Delay1/1 -> Sum/3
  Gain3/1 -> Variable Transport Delay2/1
  Variable Transport Delay2/1 -> Sum/4
  Input/1 -> Variable Transport Delay/2
  Input1/1 -> Variable Transport Delay1/2
  Input2/1 -> Variable Transport Delay2/2

== system Model_10_1/26_12_theta1 bang 0 n1=5; n2=1 /PSO-ETM5 ==
  In1 : Inport
  Input : Inport  Port=2
  Input1 : Inport  Port=3
  Input2 : Inport  Port=4
  Gain : Gain  Gain=0.1667
  Gain1 : Gain  Gain=0.3333
  Gain2 : Gain  Gain=0.3333
  Gain3 : Gain  Gain=0.1667
  Sum : Sum  Inputs=++++
  Variable Transport Delay : VariableTransportDelay  VariableDelayType=Variable transport delay  MaximumDelay=10
  Variable Transport Delay1 : VariableTransportDelay  VariableDelayType=Variable transport delay  MaximumDelay=10
  Variable Transport Delay2 : VariableTransportDelay  VariableDelayType=Variable transport delay  MaximumDelay=10
  Out1 : Outport
  wires:
  In1/1 -> Gain1/1, Gain3/1, Gain2/1, Gain/1
  Gain1/1 -> Variable Transport Delay/1
  Variable Transport Delay/1 -> Sum/2
  Sum/1 -> Out1/1
  Gain2/1 -> Variable Transport Delay1/1
  Gain/1 -> Sum/1
  Variable Transport Delay1/1 -> Sum/3
  Gain3/1 -> Variable Transport Delay2/1
  Variable Transport Delay2/1 -> Sum/4
  Input/1 -> Variable Transport Delay/2
  Input1/1 -> Variable Transport Delay1/2
  Input2/1 -> Variable Transport Delay2/2

== system Model_10_1/26_12_theta1 bang 0 n1=5; n2=1 /PSO-ETM6 ==
  In1 : Inport
  Input : Inport  Port=2
  Input1 : Inport  Port=3
  Input2 : Inport  Port=4
  Gain : Gain  Gain=0.1667
  Gain1 : Gain  Gain=0.3333
  Gain2 : Gain  Gain=0.3333
  Gain3 : Gain  Gain=0.1667
  Sum : Sum  Inputs=++++
  Variable Transport Delay : VariableTransportDelay  VariableDelayType=Variable transport delay  MaximumDelay=10
  Variable Transport Delay1 : VariableTransportDelay  VariableDelayType=Variable transport delay  MaximumDelay=10
  Variable Transport Delay2 : VariableTransportDelay  VariableDelayType=Variable transport delay  MaximumDelay=10
  ref : Outport
  wires:
  In1/1 -> Gain1/1, Gain3/1, Gain2/1, Gain/1
  Gain1/1 -> Variable Transport Delay/1
  Variable Transport Delay/1 -> Sum/2
  Sum/1 -> ref/1
  Gain2/1 -> Variable Transport Delay1/1
  Gain/1 -> Sum/1
  Variable Transport Delay1/1 -> Sum/3
  Gain3/1 -> Variable Transport Delay2/1
  Variable Transport Delay2/1 -> Sum/4
  Input/1 -> Variable Transport Delay/2
  Input1/1 -> Variable Transport Delay1/2
  Input2/1 -> Variable Transport Delay2/2

== system Model_10_1/26_12_theta1 bang 0 n1=5; n2=1 /PSO-ETM7 ==
  In1 : Inport
  Input : Inport  Port=2
  Input1 : Inport  Port=3
  Input2 : Inport  Port=4
  Gain : Gain  Gain=A1_etm4_2
  Gain1 : Gain  Gain=A2_etm4_2
  Gain2 : Gain  Gain=A3_etm4_2
  Gain3 : Gain  Gain=A4_etm4_2
  Sum : Sum  Inputs=++++
  Variable Transport Delay : VariableTransportDelay  VariableDelayType=Variable transport delay  MaximumDelay=10
  Variable Transport Delay1 : VariableTransportDelay  VariableDelayType=Variable transport delay  MaximumDelay=10
  Variable Transport Delay2 : VariableTransportDelay  VariableDelayType=Variable transport delay  MaximumDelay=10
  ref : Outport
  wires:
  In1/1 -> Gain1/1, Gain3/1, Gain2/1, Gain/1
  Gain1/1 -> Variable Transport Delay/1
  Variable Transport Delay/1 -> Sum/2
  Sum/1 -> ref/1
  Gain2/1 -> Variable Transport Delay1/1
  Gain/1 -> Sum/1
  Variable Transport Delay1/1 -> Sum/3
  Gain3/1 -> Variable Transport Delay2/1
  Variable Transport Delay2/1 -> Sum/4
  Input/1 -> Variable Transport Delay/2
  Input1/1 -> Variable Transport Delay1/2
  Input2/1 -> Variable Transport Delay2/2

== system Model_10_1/26_12_theta1 bang 0 n1=5; n2=1 /PSO-ETM8 ==
  In1 : Inport
  Input : Inport  Port=2
  Input1 : Inport  Port=3
  Input2 : Inport  Port=4
  Gain : Gain  Gain=0.1667
  Gain1 : Gain  Gain=0.3333
  Gain2 : Gain  Gain=0.3333
  Gain3 : Gain  Gain=0.1667
  Sum : Sum  Inputs=++++
  Variable Transport Delay : VariableTransportDelay  VariableDelayType=Variable transport delay  MaximumDelay=10
  Variable Transport Delay1 : VariableTransportDelay  VariableDelayType=Variable transport delay  MaximumDelay=10
  Variable Transport Delay2 : VariableTransportDelay  VariableDelayType=Variable transport delay  MaximumDelay=10
  ref : Outport
  wires:
  In1/1 -> Gain1/1, Gain3/1, Gain2/1, Gain/1
  Gain1/1 -> Variable Transport Delay/1
  Variable Transport Delay/1 -> Sum/2
  Sum/1 -> ref/1
  Gain2/1 -> Variable Transport Delay1/1
  Gain/1 -> Sum/1
  Variable Transport Delay1/1 -> Sum/3
  Gain3/1 -> Variable Transport Delay2/1
  Variable Transport Delay2/1 -> Sum/4
  Input/1 -> Variable Transport Delay/2
  Input1/1 -> Variable Transport Delay1/2
  Input2/1 -> Variable Transport Delay2/2

== system Model_10_1/26_12_theta1 bang 0 n1=5; n2=1 /PSO-ETM9 ==
  In1 : Inport
  Input : Inport  Port=2
  Input1 : Inport  Port=3
  Input2 : Inport  Port=4
  Gain : Gain  Gain=0.1667
  Gain1 : Gain  Gain=0.3333
  Gain2 : Gain  Gain=0.3333
  Gain3 : Gain  Gain=0.1667
  Sum : Sum  Inputs=++++
  Variable Transport Delay : VariableTransportDelay  VariableDelayType=Variable transport delay  MaximumDelay=10
  Variable Transport Delay1 : VariableTransportDelay  VariableDelayType=Variable transport delay  MaximumDelay=10
  Variable Transport Delay2 : VariableTransportDelay  VariableDelayType=Variable transport delay  MaximumDelay=10
  ref : Outport
  wires:
  In1/1 -> Gain1/1, Gain3/1, Gain2/1, Gain/1
  Gain1/1 -> Variable Transport Delay/1
  Variable Transport Delay/1 -> Sum/2
  Sum/1 -> ref/1
  Gain2/1 -> Variable Transport Delay1/1
  Gain/1 -> Sum/1
  Variable Transport Delay1/1 -> Sum/3
  Gain3/1 -> Variable Transport Delay2/1
  Variable Transport Delay2/1 -> Sum/4
  Input/1 -> Variable Transport Delay/2
  Input1/1 -> Variable Transport Delay1/2
  Input2/1 -> Variable Transport Delay2/2

== system Model_10_1/26_12_theta1 bang 0 n1=5; n2=1 /Radial Basis Network1 ==
  Input : Inport  PortDimensions=2
      mask Display: e = 0.06;c1 = [120 230 180]/255;c2 = ([120 230 180]+0)/(256+128);c3 = ([120 230 180]+128)/(256+128);patch([0 1 1 0],[0 0 1 1],c1);patch([0 1 1 1-e 1-e 0+e],[0 0 1 1-e 0+e 0+e],c2);patch([0 0 1 1-e 0+e 0+e],[0 1 1 1-e 1-e 0+e],c3);plot([0 1 1 0 0],[0 0 1 1 0]);
  Layer 1 : Subsystem
      mask Display: e = 0.06;c1 = [120 150 230]/255;c2 = ([120 150 230]+0)/383;c3 = ([120 150 230]+128)/383;patch([0 1 1 0],[0 0 1 1],c1);patch([0 1 1 1-e 1-e 0+e],[0 0 1 1-e 0+e 0+e],c2);patch([0 0 1 1-e 0+e 0+e],[0 1 1 1-e 1-e 0+e],c3);plot([0 1 1 0 0],[0 0 1 1 0]);
  Layer 2 : Subsystem
      mask Display: e = 0.06;c1 = [120 150 230]/255;c2 = ([120 150 230]+0)/383;c3 = ([120 150 230]+128)/383;patch([0 1 1 0],[0 0 1 1],c1);patch([0 1 1 1-e 1-e 0+e],[0 0 1 1-e 0+e 0+e],c2);patch([0 0 1 1-e 0+e 0+e],[0 1 1 1-e 1-e 0+e],c3);plot([0 1 1 0 0],[0 0 1 1 0]);
  Process Input 1 : Subsystem
      mask Display: e = 0.06;c1 = [120 150 230]/255;c2 = ([120 150 230]+0)/383;c3 = ([120 150 230]+128)/383;patch([0 1 1 0],[0 0 1 1],c1);patch([0 1 1 1-e 1-e 0+e],[0 0 1 1-e 0+e 0+e],c2);patch([0 0 1 1-e 0+e 0+e],[0 1 1 1-e 1-e 0+e],c3);plot([0 1 1 0 0],[0 0 1 1 0]);
  Process Output 1 : Subsystem
      mask Display: e = 0.06;c1 = [120 150 230]/255;c2 = ([120 150 230]+0)/383;c3 = ([120 150 230]+128)/383;patch([0 1 1 0],[0 0 1 1],c1);patch([0 1 1 1-e 1-e 0+e],[0 0 1 1-e 0+e 0+e],c2);patch([0 0 1 1-e 0+e 0+e],[0 1 1 1-e 1-e 0+e],c3);plot([0 1 1 0 0],[0 0 1 1 0]);
  Output : Outport  InitialOutput=[0;0;0]
      mask Display: e = 0.06;c1 = [120 230 180]/255;c2 = ([120 230 180]+0)/(256+128);c3 = ([120 230 180]+128)/(256+128);patch([0 1 1 0],[0 0 1 1],c1);patch([0 1 1 1-e 1-e 0+e],[0 0 1 1-e 0+e 0+e],c2);patch([0 0 1 1-e 0+e 0+e],[0 1 1 1-e 1-e 0+e],c3);plot([0 1 1 0 0],[0 0 1 1 0]);
  wires:
  Input/1 -> Process Input 1/1(x)
  Process Output 1/1(y) -> Output/1
  Process Input 1/1(p) -> Layer 1/1("p{1}")
  Layer 1/1("a{1}") -> [feedback1]
  [feedback1] -> Layer 2/1("a{1} ")
  Layer 2/1("a{2}") -> Process Output 1/1(a)

== system Model_10_1/26_12_theta1 bang 0 n1=5; n2=1 /Subsystem1 ==
  e : Inport
  e1 : Inport  Port=2
  Display : Display
  Display12 : Display
  Display16 : Display
  Fitness APS 1 : Subsystem
  Fitness APS 2 : Subsystem
  Gain : Gain  Gain=n1
  Gain19 : Gain  Gain=n2
  Gain20 : Gain  Gain=n2
  Scope : Scope
  Scope71 : Scope
  Scope72 : Scope
  Subtract : Sum
  Subtract1 : Sum  Inputs=+++
  Out1 : Outport
  wires:
  Fitness APS 2/2(MAx) -> Gain20/1, Display16/1, Scope71/1
  Fitness APS 1/2(MAx) -> Display12/1, Gain19/1, Scope72/1
  Subtract/1 -> Gain/1, Display/1, Scope/1
  Gain20/1 -> Subtract1/3
  e/1 -> Fitness APS 1/1(e)
  Gain/1 -> Subtract1/1
  Fitness APS 1/1(IAE) -> Subtract/1
  Gain19/1 -> Subtract1/2
  Fitness APS 2/1(IAE) -> Subtract/2
  e1/1 -> Fitness APS 2/1(e)
  Subtract1/1 -> Out1/1

== system Model_10_1/26_12_theta1 bang 0 n1=5; n2=1 /Subsystem2 ==
  e : Inport
  e1 : Inport  Port=2
  Display : Display
  Display12 : Display
  Display16 : Display
  Fitness APS 1 : Subsystem
  Fitness APS 2 : Subsystem
  Gain : Gain  Gain=n1
  Gain19 : Gain  Gain=n2
  Gain20 : Gain  Gain=n2
  Scope : Scope
  Scope71 : Scope
  Scope72 : Scope
  Subtract : Sum
  Subtract1 : Sum  Inputs=+++
  Out1 : Outport
  wires:
  Fitness APS 2/2(MAx) -> Gain20/1, Display16/1, Scope71/1
  Fitness APS 1/2(MAx) -> Display12/1, Gain19/1, Scope72/1
  Subtract/1 -> Gain/1, Display/1, Scope/1
  Gain20/1 -> Subtract1/3
  e/1 -> Fitness APS 1/1(e)
  Gain/1 -> Subtract1/1
  Fitness APS 1/1(IAE) -> Subtract/1
  Gain19/1 -> Subtract1/2
  Fitness APS 2/1(IAE) -> Subtract/2
  e1/1 -> Fitness APS 2/1(e)
  Subtract1/1 -> Out1/1

== system Model_10_1/26_12_theta1 bang 0 n1=5; n2=1 /Subsystem3 ==
  e : Inport
  e1 : Inport  Port=2
  Display : Display
  Display12 : Display
  Display16 : Display
  Fitness APS 1 : Subsystem
  Fitness APS 2 : Subsystem
  Gain : Gain  Gain=n1
  Gain19 : Gain  Gain=n2
  Gain20 : Gain  Gain=n2
  Scope : Scope
  Scope71 : Scope
  Scope72 : Scope
  Subtract : Sum
  Subtract1 : Sum  Inputs=+++
  Out1 : Outport
  wires:
  Fitness APS 2/2(MAx) -> Gain20/1, Display16/1, Scope71/1
  Fitness APS 1/2(MAx) -> Display12/1, Gain19/1, Scope72/1
  Subtract/1 -> Gain/1, Display/1, Scope/1
  Gain20/1 -> Subtract1/3
  e/1 -> Fitness APS 1/1(e)
  Gain/1 -> Subtract1/1
  Fitness APS 1/1(IAE) -> Subtract/1
  Gain19/1 -> Subtract1/2
  Fitness APS 2/1(IAE) -> Subtract/2
  e1/1 -> Fitness APS 2/1(e)
  Subtract1/1 -> Out1/1

== system Model_10_1/26_12_theta1 bang 0 n1=5; n2=1 /Subsystem4 ==
  e : Inport
  e1 : Inport  Port=2
  Display : Display
  Display12 : Display
  Display16 : Display
  Fitness APS 1 : Subsystem
  Fitness APS 2 : Subsystem
  Gain : Gain  Gain=n1
  Gain19 : Gain  Gain=n2
  Gain20 : Gain  Gain=n2
  Scope : Scope
  Scope71 : Scope
  Scope72 : Scope
  Subtract : Sum
  Subtract1 : Sum  Inputs=+++
  Out1 : Outport
  wires:
  Fitness APS 2/2(MAx) -> Gain20/1, Display16/1, Scope71/1
  Fitness APS 1/2(MAx) -> Display12/1, Gain19/1, Scope72/1
  Subtract/1 -> Gain/1, Display/1, Scope/1
  Gain20/1 -> Subtract1/3
  e/1 -> Fitness APS 1/1(e)
  Gain/1 -> Subtract1/1
  Fitness APS 1/1(IAE) -> Subtract/1
  Gain19/1 -> Subtract1/2
  Fitness APS 2/1(IAE) -> Subtract/2
  e1/1 -> Fitness APS 2/1(e)
  Subtract1/1 -> Out1/1

== system Model_10_1/26_12_theta1 bang 0 n1=5; n2=1 /Subsystem5 ==
  e : Inport
  e1 : Inport  Port=2
  Display : Display
  Display12 : Display
  Display16 : Display
  Fitness APS 1 : Subsystem
  Fitness APS 2 : Subsystem
  Gain : Gain  Gain=n1
  Gain19 : Gain  Gain=n2
  Gain20 : Gain  Gain=n2
  Scope : Scope
  Scope71 : Scope
  Scope72 : Scope
  Subtract : Sum
  Subtract1 : Sum  Inputs=+++
  Out1 : Outport
  wires:
  Fitness APS 2/2(MAx) -> Gain20/1, Display16/1, Scope71/1
  Fitness APS 1/2(MAx) -> Display12/1, Gain19/1, Scope72/1
  Subtract/1 -> Gain/1, Display/1, Scope/1
  Gain20/1 -> Subtract1/3
  e/1 -> Fitness APS 1/1(e)
  Gain/1 -> Subtract1/1
  Fitness APS 1/1(IAE) -> Subtract/1
  Gain19/1 -> Subtract1/2
  Fitness APS 2/1(IAE) -> Subtract/2
  e1/1 -> Fitness APS 2/1(e)
  Subtract1/1 -> Out1/1

== system Model_10_1/26_12_theta1 bang 0 n1=5; n2=1 /Subsystem6 ==
  e : Inport
  e1 : Inport  Port=2
  Display : Display
  Display12 : Display
  Display16 : Display
  Fitness APS 1 : Subsystem
  Fitness APS 2 : Subsystem
  Gain : Gain  Gain=n1
  Gain19 : Gain  Gain=n2
  Gain20 : Gain  Gain=n2
  Scope : Scope
  Scope71 : Scope
  Scope72 : Scope
  Subtract : Sum
  Subtract1 : Sum  Inputs=+++
  Out1 : Outport
  wires:
  Fitness APS 2/2(MAx) -> Gain20/1, Display16/1, Scope71/1
  Fitness APS 1/2(MAx) -> Display12/1, Gain19/1, Scope72/1
  Subtract/1 -> Gain/1, Display/1, Scope/1
  Gain20/1 -> Subtract1/3
  e/1 -> Fitness APS 1/1(e)
  Gain/1 -> Subtract1/1
  Fitness APS 1/1(IAE) -> Subtract/1
  Gain19/1 -> Subtract1/2
  Fitness APS 2/1(IAE) -> Subtract/2
  e1/1 -> Fitness APS 2/1(e)
  Subtract1/1 -> Out1/1

== system Model_10_1/26_12_theta1 bang 0 n1=5; n2=1 /ban đầu theta1=5pi//180, theta2=3pi//180_1 ==
  Fx : Inport
  Fl : Inport  Port=2
  Add : Sum
  Constant : Constant  Value=-(m1+mc)*g
  Constant1 : Constant  Value=mc
  Constant2 : Constant  Value=L_tai
  Crane : MATLAB Function  TreatAsAtomicUnit=on
  Integrator{,1,3,5,7} (5 alike) : Integrator
  Integrator2 : Integrator  InitialCondition=l
  Integrator4 : Integrator  InitialCondition=theta1_ini
  Integrator6 : Integrator  InitialCondition=theta2_ini
  Scope{1..5} (5 alike) : Scope
  x : Outport
  l : Outport  Port=2
  the1 : Outport  Port=3
  the2 : Outport  Port=4
  wires:
  Integrator5/1 -> [x6]
  Integrator2/1 -> Scope4/1, l/1, [x3]
  Integrator1/1 -> [x2]
  Integrator/1 -> x/1, [x1]
  Integrator3/1 -> [x4]
  Add/1 -> Crane/9(Fl), Scope1/1
  Integrator6/1 -> Scope2/1, the2/1, [x7]
  Integrator7/1 -> [x8]
  Crane/1(dx1) -> Integrator/1
  Crane/2(dx2) -> Integrator1/1
  Crane/3(dx3) -> Integrator2/1
  Crane/4(dx4) -> Integrator3/1
  Crane/5(dx5) -> Integrator4/1
  Crane/6(dx6) -> Integrator5/1
  Crane/7(dx7) -> Integrator6/1
  Crane/8(dx8) -> Integrator7/1
  Fx/1 -> Crane/8(Fx)
  Constant1/1 -> Crane/10(m2)
  [x2] -> Crane/1(d1x)
  [x3] -> Crane/2(l1)
  [x4] -> Crane/3(d1l1)
  [x5] -> Crane/4(the1)
  [x6] -> Crane/5(d1the1)
  [x7] -> Crane/6(the2)
  [x8] -> Crane/7(d1the2)
  Integrator4/1 -> Scope3/1, the1/1, [x5]
  Fl/1 -> Add/2
  [x1] -> Scope5/1
  Constant/1 -> Add/1
  Constant2/1 -> Crane/11(l2)

== system Model_10_1/26_12_theta1 bang 0 n1=5; n2=1 /ban đầu theta1=5pi//180, theta2=3pi//180_2 ==
  Fx : Inport
  Fl : Inport  Port=2
  Add : Sum
  Constant : Constant  Value=-(m1+mc)*g
  Constant1 : Constant  Value=mc
  Constant2 : Constant  Value=L_tai
  Crane : MATLAB Function  TreatAsAtomicUnit=on
  Integrator{,1,3,5,7} (5 alike) : Integrator
  Integrator2 : Integrator  InitialCondition=l
  Integrator4 : Integrator  InitialCondition=theta1_ini
  Integrator6 : Integrator  InitialCondition=theta2_ini
  Scope{1..5} (5 alike) : Scope
  x : Outport
  l : Outport  Port=2
  the1 : Outport  Port=3
  the2 : Outport  Port=4
  wires:
  Integrator5/1 -> [x6]
  Integrator2/1 -> Scope4/1, l/1, [x3]
  Integrator1/1 -> [x2]
  Integrator/1 -> x/1, [x1]
  Integrator3/1 -> [x4]
  Add/1 -> Crane/9(Fl), Scope1/1
  Integrator6/1 -> Scope2/1, the2/1, [x7]
  Integrator7/1 -> [x8]
  Crane/1(dx1) -> Integrator/1
  Crane/2(dx2) -> Integrator1/1
  Crane/3(dx3) -> Integrator2/1
  Crane/4(dx4) -> Integrator3/1
  Crane/5(dx5) -> Integrator4/1
  Crane/6(dx6) -> Integrator5/1
  Crane/7(dx7) -> Integrator6/1
  Crane/8(dx8) -> Integrator7/1
  Fx/1 -> Crane/8(Fx)
  Constant1/1 -> Crane/10(m2)
  [x2] -> Crane/1(d1x)
  [x3] -> Crane/2(l1)
  [x4] -> Crane/3(d1l1)
  [x5] -> Crane/4(the1)
  [x6] -> Crane/5(d1the1)
  [x7] -> Crane/6(the2)
  [x8] -> Crane/7(d1the2)
  Integrator4/1 -> Scope3/1, the1/1, [x5]
  Fl/1 -> Add/2
  [x1] -> Scope5/1
  Constant/1 -> Add/1
  Constant2/1 -> Crane/11(l2)

== system Model_10_1/26_12_theta1 bang 0 n1=5; n2=1 /ban đầu theta1=5pi//180, theta2=3pi//180_3 ==
  Fx : Inport
  Fl : Inport  Port=2
  Add : Sum
  Constant : Constant  Value=-(m1+mc)*g
  Constant1 : Constant  Value=mc
  Constant2 : Constant  Value=L_tai
  Crane : MATLAB Function  TreatAsAtomicUnit=on
  Integrator{,1,3,5,7} (5 alike) : Integrator
  Integrator2 : Integrator  InitialCondition=l
  Integrator4 : Integrator  InitialCondition=theta1_ini
  Integrator6 : Integrator  InitialCondition=theta2_ini
  Scope{1..5} (5 alike) : Scope
  x : Outport
  l : Outport  Port=2
  the1 : Outport  Port=3
  the2 : Outport  Port=4
  wires:
  Integrator5/1 -> [x6]
  Integrator2/1 -> Scope4/1, l/1, [x3]
  Integrator1/1 -> [x2]
  Integrator/1 -> x/1, [x1]
  Integrator3/1 -> [x4]
  Add/1 -> Crane/9(Fl), Scope1/1
  Integrator6/1 -> Scope2/1, the2/1, [x7]
  Integrator7/1 -> [x8]
  Crane/1(dx1) -> Integrator/1
  Crane/2(dx2) -> Integrator1/1
  Crane/3(dx3) -> Integrator2/1
  Crane/4(dx4) -> Integrator3/1
  Crane/5(dx5) -> Integrator4/1
  Crane/6(dx6) -> Integrator5/1
  Crane/7(dx7) -> Integrator6/1
  Crane/8(dx8) -> Integrator7/1
  Fx/1 -> Crane/8(Fx)
  Constant1/1 -> Crane/10(m2)
  [x2] -> Crane/1(d1x)
  [x3] -> Crane/2(l1)
  [x4] -> Crane/3(d1l1)
  [x5] -> Crane/4(the1)
  [x6] -> Crane/5(d1the1)
  [x7] -> Crane/6(the2)
  [x8] -> Crane/7(d1the2)
  Integrator4/1 -> Scope3/1, the1/1, [x5]
  Fl/1 -> Add/2
  [x1] -> Scope5/1
  Constant/1 -> Add/1
  Constant2/1 -> Crane/11(l2)

== system Model_10_1/26_12_theta1 bang 0 n1=5; n2=1 /ban đầu theta1=5pi//180, theta2=3pi//180_4 ==
  Fx : Inport
  Fl : Inport  Port=2
  Add : Sum
  Constant : Constant  Value=-(m1+mc)*g
  Constant1 : Constant  Value=mc
  Constant2 : Constant  Value=L_tai
  Crane : MATLAB Function  TreatAsAtomicUnit=on
  Integrator{,1,3,5,7} (5 alike) : Integrator
  Integrator2 : Integrator  InitialCondition=l
  Integrator4 : Integrator  InitialCondition=theta1_ini
  Integrator6 : Integrator  InitialCondition=theta2_ini
  Scope{1..5} (5 alike) : Scope
  x : Outport
  l : Outport  Port=2
  the1 : Outport  Port=3
  the2 : Outport  Port=4
  wires:
  Integrator5/1 -> [x6]
  Integrator2/1 -> Scope4/1, l/1, [x3]
  Integrator1/1 -> [x2]
  Integrator/1 -> x/1, [x1]
  Integrator3/1 -> [x4]
  Add/1 -> Crane/9(Fl), Scope1/1
  Integrator6/1 -> Scope2/1, the2/1, [x7]
  Integrator7/1 -> [x8]
  Crane/1(dx1) -> Integrator/1
  Crane/2(dx2) -> Integrator1/1
  Crane/3(dx3) -> Integrator2/1
  Crane/4(dx4) -> Integrator3/1
  Crane/5(dx5) -> Integrator4/1
  Crane/6(dx6) -> Integrator5/1
  Crane/7(dx7) -> Integrator6/1
  Crane/8(dx8) -> Integrator7/1
  Fx/1 -> Crane/8(Fx)
  Constant1/1 -> Crane/10(m2)
  [x2] -> Crane/1(d1x)
  [x3] -> Crane/2(l1)
  [x4] -> Crane/3(d1l1)
  [x5] -> Crane/4(the1)
  [x6] -> Crane/5(d1the1)
  [x7] -> Crane/6(the2)
  [x8] -> Crane/7(d1the2)
  Integrator4/1 -> Scope3/1, the1/1, [x5]
  Fl/1 -> Add/2
  [x1] -> Scope5/1
  Constant/1 -> Add/1
  Constant2/1 -> Crane/11(l2)
